simulink model "encoder"  (R2024b)
settings: Solver=FixedStepAuto  StartTime=0.0  StopTime=inf  FixedStep=0.1  RelTol=1e-3  EnableMultiTasking=on
libraries: stm32g4xxblockslib x3, stm32f4xxblockslib x2
settings Model: STM32="{\"EncoderBlockForG4\":[{\"ID\":\"encoder:1\"},{\"ID\":\"encoder:37\"},{\"ID\":\"encoder:57\"}],\"DigitalPortRead\":[{\"ID\":\"encoder:14\"},{\"ID\":\"encoder:63\"}]}"  Creator=janej  LastModifiedBy=janej
settings OptimizationCC: DefaultParameterBehavior=Inlined  EnhancedBackFolding=on  PassReuseOutputArgsAs=Individual arguments  ZeroExternalMemoryAtStartup=off  ZeroInternalMemoryAtStartup=off  MaxStackSize=512  OptimizeBlockOrder=speed  DifferentSizesBufferReuse=on  OptimizationCustomize=off  EfficientTunableParamExpr=on
settings DebuggingCC: ParameterTunabilityLossMsg=error
settings HardwareCC: ProdBitPerPointer=32  ProdBitPerSizeT=32  ProdBitPerPtrDiffT=32  ProdLargestAtomicInteger=Long  ProdLargestAtomicFloat=Double  ProdWordSize=32  ProdLongLongMode=on  ProdHWDeviceType=ARM Compatible->ARM Cortex-M
settings SFSimCC: MATLABDynamicMemAlloc=off
settings RTWCC: Description=Embedded Coder  SystemTargetFile=ert.tlc  HardwareBoard=STM32G4xx Based  TemplateMakefile=ert_default_tmf  Toolchain=GNU Tools for ARM Embedded Processors
settings CodeAppCC: ForceParamTrailComments=on  IgnoreCustomStorageClasses=off  OperatorAnnotations=on  SimulinkDataObjDesc=on  SFDataObjDesc=on  InsertBlockDesc=on
settings ERTTargetCC: TargetLangStandard=C99 (ISO)  CodeReplacementLibrary=ARM Cortex-M  ExtModeTransport=3  ExtModeStaticAlloc=on  ExtModeStaticAllocSize=2048  ExtModeMexFile=ext_xcp  ExtModeIntrfLevel=Level2 - Open

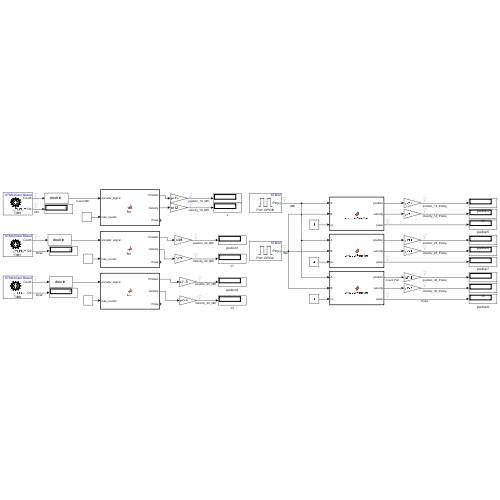
[thumbnail: Simulink's stored preview of the top-level diagram]
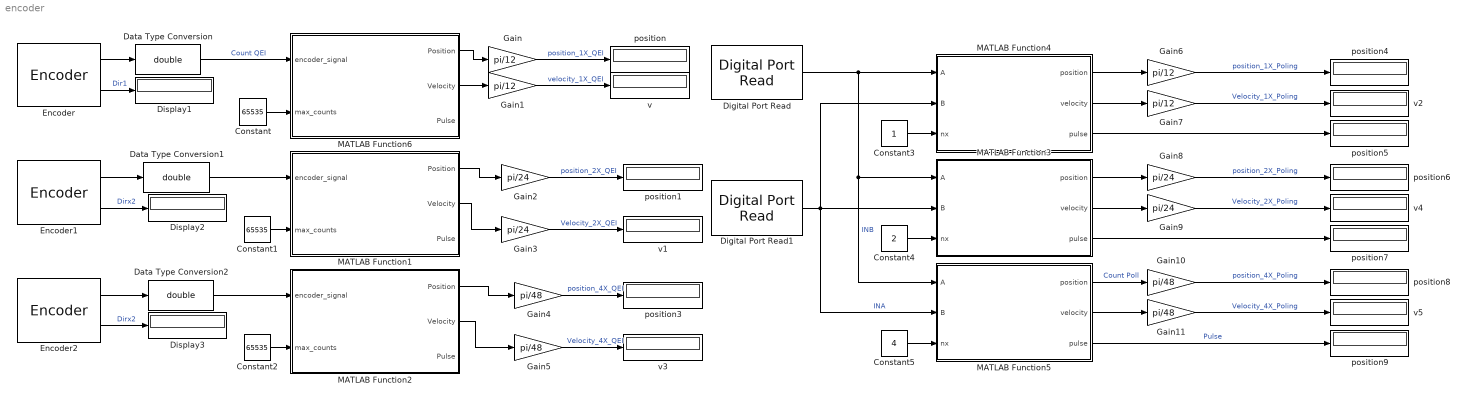
== system encoder ==
  Constant : Constant  Value=65535
  Constant1 : Constant  Value=65535
  Constant2 : Constant  Value=65535
  Constant3 : Constant
  Constant4 : Constant  Value=2
  Constant5 : Constant  Value=4
  Data Type Conversion : DataTypeConversion  OutDataTypeStr=double  SaturateOnIntegerOverflow=off  RndMeth=Floor
  Data Type Conversion1 : DataTypeConversion  OutDataTypeStr=double  SaturateOnIntegerOverflow=off  RndMeth=Floor
  Data Type Conversion2 : DataTypeConversion  OutDataTypeStr=double  SaturateOnIntegerOverflow=off  RndMeth=Floor
  Digital Port Read : stm32f4xxblockslib/Digital Port Read  PortName=GPIOB  PinNumber=[10]  ReadOperation=on  IOAsArray=on  SampleTime=-1  EnableSimPort=off  hoistedMaskSrc=ECSoC/ECSimCodegen/Digital Port Read
      settings: LibrarySourceBlock=stm32g4xxblockslib/Digital Port Read
  Digital Port Read1 : stm32f4xxblockslib/Digital Port Read  PortName=GPIOA  PinNumber=[8]  ReadOperation=on  IOAsArray=on  SampleTime=-1  EnableSimPort=off  hoistedMaskSrc=ECSoC/ECSimCodegen/Digital Port Read
      settings: LibrarySourceBlock=stm32g4xxblockslib/Digital Port Read
  Display1 : Display
  Display2 : Display
  Display3 : Display
  Encoder : stm32g4xxblockslib/Encoder  TimerModule=TIM3  EnableResetInput=off  OutputCountAfterFirstIndex=off  OutputValidIndex=off  OutputDirection=on  OutputStatus=off  SampleTime=-1
  Encoder1 : stm32g4xxblockslib/Encoder  TimerModule=TIM1  EnableResetInput=off  OutputCountAfterFirstIndex=off  OutputValidIndex=off  OutputDirection=on  OutputStatus=off  SampleTime=-1
  Encoder2 : stm32g4xxblockslib/Encoder  TimerModule=TIM8  EnableResetInput=off  OutputCountAfterFirstIndex=off  OutputValidIndex=off  OutputDirection=on  OutputStatus=off  SampleTime=-1
  Gain{,1,6..7} (4 alike) : Gain  Gain=pi/12
  Gain{4..5,10..11} (4 alike) : Gain  Gain=pi/48
  Gain{2..3,8..9} (4 alike) : Gain  Gain=pi/24
  MATLAB Function1 : MATLAB Function  TreatAsAtomicUnit=on
  MATLAB Function2 : MATLAB Function  TreatAsAtomicUnit=on
  MATLAB Function3 : MATLAB Function  TreatAsAtomicUnit=on
  MATLAB Function4 : MATLAB Function  TreatAsAtomicUnit=on
  MATLAB Function5 : MATLAB Function  TreatAsAtomicUnit=on
  MATLAB Function6 : MATLAB Function  TreatAsAtomicUnit=on
  position{,1,3..9} (9 alike) : Display
  v{,1..5} (6 alike) : Display
  wires:
  Encoder/2 -> Display1/1  "Dir1"
  Encoder/1 -> Data Type Conversion/1
  Data Type Conversion/1 -> MATLAB Function6/1(encoder_signal)  "Count QEI"
  Constant/1 -> MATLAB Function6/2(max_counts)
  Gain/1 -> position/1  "position_1X_QEI"
  Gain1/1 -> v/1  "velocity_1X_QEI"
  Gain3/1 -> v1/1  "Velocity_2X_QEI"
  Gain2/1 -> position1/1  "position_2X_QEI"
  MATLAB Function1/2(Velocity) -> Gain3/1
  Constant1/1 -> MATLAB Function1/2(max_counts)
  Data Type Conversion1/1 -> MATLAB Function1/1(encoder_signal)
  Encoder1/1 -> Data Type Conversion1/1
  MATLAB Function1/1(Position) -> Gain2/1
  Encoder1/2 -> Display2/1  "Dirx2"
  Encoder2/2 -> Display3/1  "Dirx2"
  MATLAB Function2/1(Position) -> Gain4/1
  Encoder2/1 -> Data Type Conversion2/1
  Data Type Conversion2/1 -> MATLAB Function2/1(encoder_signal)
  Constant2/1 -> MATLAB Function2/2(max_counts)
  MATLAB Function2/2(Velocity) -> Gain5/1
  Gain4/1 -> position3/1  "position_4X_QEI"
  Gain5/1 -> v3/1  "Velocity_4X_QEI"
  Digital Port Read/1 -> MATLAB Function4/1(A), MATLAB Function3/1(A), MATLAB Function5/1(A)  "INB"
  Constant3/1 -> MATLAB Function4/3(nx)
  MATLAB Function4/1(position) -> Gain6/1
  MATLAB Function4/2(velocity) -> Gain7/1
  MATLAB Function4/3(pulse) -> position5/1
  Digital Port Read1/1 -> MATLAB Function4/2(B), MATLAB Function3/2(B), MATLAB Function5/2(B)  "INA"
  MATLAB Function3/2(velocity) -> Gain9/1
  MATLAB Function3/1(position) -> Gain8/1
  MATLAB Function3/3(pulse) -> position7/1
  Constant4/1 -> MATLAB Function3/3(nx)
  MATLAB Function5/2(velocity) -> Gain11/1
  MATLAB Function5/1(position) -> Gain10/1  "Count Poll"
  MATLAB Function5/3(pulse) -> position9/1  "Pulse"
  Constant5/1 -> MATLAB Function5/3(nx)
  Gain6/1 -> position4/1  "position_1X_Poling"
  Gain7/1 -> v2/1  "Velocity_1X_Poling"
  Gain8/1 -> position6/1  "position_2X_Poling"
  Gain9/1 -> v4/1  "Velocity_2X_Poling"
  Gain11/1 -> v5/1  "Velocity_4X_Poling"
  Gain10/1 -> position8/1  "position_4X_Poling"
  MATLAB Function6/1(Position) -> Gain/1
  MATLAB Function6/2(Velocity) -> Gain1/1

== matlab function encoder/MATLAB Function1 ==
  data: encoder_signal input; Position output; Velocity output; max_counts input; Pulse output
function [Position, Velocity, Pulse] = fcn(encoder_signal, max_counts)

    persistent prev_signal corrected_sum;
    if isempty(prev_signal)
        prev_signal = encoder_signal;
        corrected_sum = encoder_signal;
    end
    Velocity = 0;
    delta = encoder_signal - prev_signal;

    if delta < -max_counts / 2
        corrected_sum = corrected_sum + (delta + max_counts);
    elseif delta > max_counts / 2
        corrected_sum = corrected_sum + (delta - max_counts);
    else
        corrected_sum = corrected_sum + delta;
        dt = 0.1;  
        Velocity = delta / dt;
    end

    prev_signal = encoder_signal;

    Position = corrected_sum;
    Pulse = encoder_signal;
end

== matlab function encoder/MATLAB Function2 ==
  data: encoder_signal input; Position output; Velocity output; max_counts input; Pulse output
function [Position, Velocity, Pulse] = fcn(encoder_signal, max_counts)

    persistent prev_signal corrected_sum;
    if isempty(prev_signal)
        prev_signal = encoder_signal;
        corrected_sum = encoder_signal;
    end
    Velocity = 0;
    delta = encoder_signal - prev_signal;

    if delta < -max_counts / 2
        corrected_sum = corrected_sum + (delta + max_counts);
    elseif delta > max_counts / 2
        corrected_sum = corrected_sum + (delta - max_counts);
    else
        corrected_sum = corrected_sum + delta;
        dt = 0.1;  
        Velocity = delta / dt;
    end

    prev_signal = encoder_signal;

    Position = corrected_sum;
    Pulse = encoder_signal;
end

== matlab function encoder/MATLAB Function3 ==
  data: A input; position output; B input; nx input; velocity output; pulse output
function [position, velocity, pulse] = encoderFunction(A, B, nx)
    % encoderFunction calculates position, velocity, and pulse count
    % A, B  : encoder signals (digital)
    % nx    : encoder mode (1x, 2x, or 4x)
    % position : cumulative position in counts
    % velocity : change in position (counts per time step)
    % pulse    : total pulse count (absolute value)

    % Declare persistent variables to store previous states
    persistent prevA prevB prevPosition prevTime pulseCount
    
    if isempty(prevA)
        % Initialize persistent variables on first run
        prevA = A;
        prevB = B;
        prevPosition = 0;
        prevTime = 0;
        pulseCount = 0;
    end
    
    % Calculate the direction and count based on mode (nx)
    deltaPosition = 0;
    if nx == 1
        % 1x mode: Only count on rising edges of A signal
        if A ~= prevA && A == 1  % Rising edge of A
            if B == 0
                deltaPosition = 1;
            else
                deltaPosition = -1;
            end
        end
    elseif nx == 2
        % 2x mode: Count on rising and falling edges of A signal
        if A ~= prevA
            if B == 0
                deltaPosition = 1 * sign(A - prevA);  % +1 for rising, -1 for falling
            else
                deltaPosition = -1 * sign(A - prevA);
            end
        end
    elseif nx == 4
        % 4x mode: Count on any change in A or B
        if A ~= prevA && A == 1 
            if B == 1
                deltaPosition = -1;
            end 
            if B == 0
                deltaPosition = 1;
            end
        end
        if A ~= prevA && A == 0
            if B == 1
                deltaPosition = 1;
            end 
            if B == 0
                deltaPosition = -1;
            end
        end
        if B ~= prevB && B == 1 
            if A == 1
                deltaPosition = 1;
            end 
            if A == 0
                deltaPosition = -1;
            end
        end
        if B ~= prevB && B == 0
            if A == 1
                deltaPosition = -1;
            end 
            if A == 0
                deltaPosition = 1;
            end
        end
    end

    % Update pulse count and cumulative position
    pulseCount = pulseCount + abs(deltaPosition);
    prevPosition = prevPosition + deltaPosition;
    
    % Calculate velocity
    % Use a fixed sample time (e.g., 0.001 seconds) instead of tic/toc for Simulink
    sampleTime = 0.001;  % Adjust this to match your model’s sample time
    velocity = deltaPosition / sampleTime;  % Counts per second

    % Assign outputs
    position = prevPosition;
    pulse = pulseCount;
    
    % Update previous values
    prevA = A;
    prevB = B;
end

== matlab function encoder/MATLAB Function4 ==
  data: A input; position output; B input; nx input; velocity output; pulse output
function [position, velocity, pulse] = encoderFunction(A, B, nx)
    persistent prevA prevB prevPosition prevTime pulseCount
    
    if isempty(prevA)
        prevA = A;
        prevB = B;
        prevPosition = 0;
        prevTime = 0;
        pulseCount = 0;
    end
    
    
    deltaPosition = 0;
    if nx == 1
        if A ~= prevA && A == 1  
            if B == 0
                deltaPosition = 1;
            else
                deltaPosition = -1;
            end
        end
    elseif nx == 2
        if A ~= prevA
            if B == 0
                deltaPosition = 1 * sign(A - prevA);  
            else
                deltaPosition = -1 * sign(A - prevA);
            end
        end
    elseif nx == 4
        if A ~= prevA && A == 1 
            if B == 1
                deltaPosition = -1;
            end 
            if B == 0
                deltaPosition = 1;
            end
        end
        if A ~= prevA && A == 0
            if B == 1
                deltaPosition = 1;
            end 
            if B == 0
                deltaPosition = -1;
            end
        end
        if B ~= prevB && B == 1 
            if A == 1
                deltaPosition = 1;
            end 
            if A == 0
                deltaPosition = -1;
            end
        end
        if B ~= prevB && B == 0
            if A == 1
                deltaPosition = -1;
            end 
            if A == 0
                deltaPosition = 1;
            end
        end
    end

    pulseCount = pulseCount + abs(deltaPosition);
    prevPosition = prevPosition + deltaPosition;

    velocity = deltaPosition / sampleTime;  

    position = prevPosition;
    pulse = pulseCount;
    
    prevA = A;
    prevB = B;
end

== matlab function encoder/MATLAB Function5 ==
  data: A input; position output; B input; nx input; velocity output; pulse output
function [position, velocity, pulse] = encoderFunction(A, B, nx)
    % encoderFunction calculates position, velocity, and pulse count
    % A, B  : encoder signals (digital)
    % nx    : encoder mode (1x, 2x, or 4x)
    % position : cumulative position in counts
    % velocity : change in position (counts per time step)
    % pulse    : total pulse count (absolute value)

    % Declare persistent variables to store previous states
    persistent prevA prevB prevPosition prevTime pulseCount
    
    if isempty(prevA)
        % Initialize persistent variables on first run
        prevA = A;
        prevB = B;
        prevPosition = 0;
        prevTime = 0;
        pulseCount = 0;
    end
    
    % Calculate the direction and count based on mode (nx)
    deltaPosition = 0;
    if nx == 1
        % 1x mode: Only count on rising edges of A signal
        if A ~= prevA && A == 1  % Rising edge of A
            if B == 0
                deltaPosition = 1;
            else
                deltaPosition = -1;
            end
        end
    elseif nx == 2
        % 2x mode: Count on rising and falling edges of A signal
        if A ~= prevA
            if B == 0
                deltaPosition = 1 * sign(A - prevA);  % +1 for rising, -1 for falling
            else
                deltaPosition = -1 * sign(A - prevA);
            end
        end
    elseif nx == 4
        % 4x mode: Count on any change in A or B
        if A ~= prevA && A == 1 
            if B == 1
                deltaPosition = -1;
            end 
            if B == 0
                deltaPosition = 1;
            end
        end
        if A ~= prevA && A == 0
            if B == 1
                deltaPosition = 1;
            end 
            if B == 0
                deltaPosition = -1;
            end
        end
        if B ~= prevB && B == 1 
            if A == 1
                deltaPosition = 1;
            end 
            if A == 0
                deltaPosition = -1;
            end
        end
        if B ~= prevB && B == 0
            if A == 1
                deltaPosition = -1;
            end 
            if A == 0
                deltaPosition = 1;
            end
        end
    end

    % Update pulse count and cumulative position
    pulseCount = pulseCount + abs(deltaPosition);
    prevPosition = prevPosition + deltaPosition;
    
    % Calculate velocity
    % Use a fixed sample time (e.g., 0.001 seconds) instead of tic/toc for Simulink
    sampleTime = 0.001;  % Adjust this to match your model’s sample time
    velocity = deltaPosition / sampleTime;  % Counts per second

    % Assign outputs
    position = prevPosition;
    pulse = pulseCount;
    
    % Update previous values
    prevA = A;
    prevB = B;
end

== matlab function encoder/MATLAB Function6 ==
  data: encoder_signal input; Position output; Velocity output; max_counts input; Pulse output
function [Position, Velocity, Pulse] = fcn(encoder_signal, max_counts)

    persistent prev_signal corrected_sum;
    if isempty(prev_signal)
        prev_signal = encoder_signal;
        corrected_sum = encoder_signal;
    end
    Velocity = 0;
    delta = encoder_signal - prev_signal;

    if delta < -max_counts / 2
        corrected_sum = corrected_sum + (delta + max_counts);
    elseif delta > max_counts / 2
        corrected_sum = corrected_sum + (delta - max_counts);
    else
        corrected_sum = corrected_sum + delta;
        dt = 0.1;  
        Velocity = delta / dt;
    end

    prev_signal = encoder_signal;

    Position = corrected_sum;
    Pulse = encoder_signal;
end
